simulink model "motion_cue"  (R2015b)
settings: Solver=VariableStepAuto  StartTime=0.0  StopTime=5  FixedStep=.001  MaxStep=.01  RelTol=1e-3
libraries: simulink x1
settings Model: Creator=brownlab  LastModifiedBy=brownlab

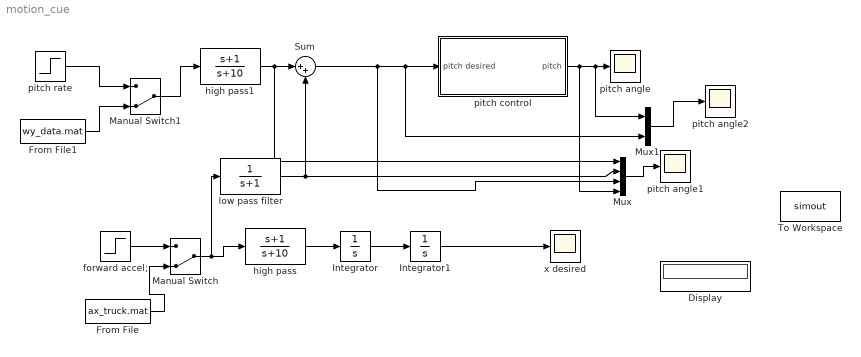
== system motion_cue ==
  Display : Display
  From File : FromFile  FileName=ax_truck.mat  SampleTime=0
  From File1 : FromFile  FileName=wy_data.mat  SampleTime=0
  Integrator : Integrator
  Integrator1 : Integrator
  Manual Switch : ManualSwitch  CurrentSetting=0
  Manual Switch1 : ManualSwitch  CurrentSetting=0
  Mux : Mux
  Mux1 : Mux  Inputs=2
  Sum : Sum  Inputs=|++
  To Workspace : ToWorkspace  VariableName=simout  SaveFormat=Timeseries  SampleTime=-1
  forward accel; : Step  SampleTime=0
  high pass : TransferFcn  Numerator=[1 1]  Denominator=[1 10]
  high pass1 : TransferFcn  Numerator=[1 1]  Denominator=[1 10]
  low pass filter : TransferFcn  Denominator=[1 1]
  pitch angle : Scope
  pitch angle1 : Scope
  pitch angle2 : Scope
  pitch control : Subsystem
  pitch rate : Step  SampleTime=0
  x desired : Scope
  wires:
  pitch control/1(pitch) -> Mux/4, Mux1/1, pitch angle/1
  high pass/1 -> Integrator/1
  Integrator/1 -> Integrator1/1
  Integrator1/1 -> x desired/1
  low pass filter/1 -> Mux/2, Sum/2
  high pass1/1 -> Mux/1, Sum/1
  Sum/1 -> Mux/3, Mux1/2, pitch control/1("pitch desired ")
  Mux/1 -> pitch angle1/1
  forward accel;/1 -> Manual Switch/1
  From File/1 -> Manual Switch/2
  Manual Switch/1 -> low pass filter/1, high pass/1
  pitch rate/1 -> Manual Switch1/1
  From File1/1 -> Manual Switch1/2
  Manual Switch1/1 -> high pass1/1
  Mux1/1 -> pitch angle2/1

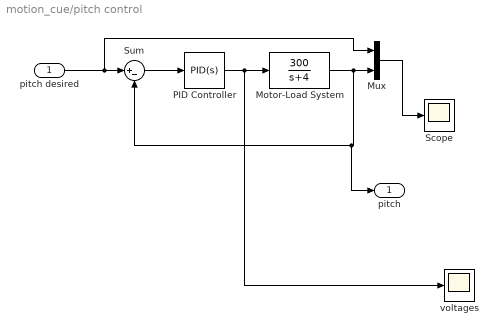
== system motion_cue/pitch control ==
  "pitch desired " : Inport
  Motor-Load System : TransferFcn  Numerator=[300]  Denominator=[1 4]
  Mux : Mux  Inputs=2
  PID Controller : simulink/Continuous/PID Controller  Controller=PID  TimeDomain=Continuous-time  SampleTime=-1  IntegratorMethod=Forward Euler  FilterMethod=Forward Euler  Form=Parallel  UseFilter=on  ControllerParametersSource=internal  P=.1  I=0  D=0  N=100  InitialConditionSource=internal  InitialConditionForIntegrator=0  InitialConditionForFilter=0  ExternalReset=none  LimitOutput=off  UpperSaturationLimit=inf  LowerSaturationLimit=-inf  LinearizeAsGain=on  AntiWindupMode=none  Kb=1  TrackingMode=off  Kt=1  PParamMin=[]  PParamMax=[]  IParamMin=[]  IParamMax=[]  DParamMin=[]  DParamMax=[]  NParamMin=[]  NParamMax=[]  KbParamMin=[]  KbParamMax=[]  KtParamMin=[]  KtParamMax=[]  POutMin=[]  POutMax=[]  IOutMin=[]  IOutMax=[]  DOutMin=[]  DOutMax=[]  NOutMin=[]  NOutMax=[]  KbOutMin=[]  KbOutMax=[]  KtOutMin=[]  KtOutMax=[]  IntegratorOutMin=[]  IntegratorOutMax=[]  FilterOutMin=[]  FilterOutMax=[]  SumOutMin=[]  SumOutMax=[]  SumI1OutMin=[]  SumI1OutMax=[]  SumI2OutMin=[]  SumI2OutMax=[]  SumI3OutMin=[]  SumI3OutMax=[]  SumDOutMin=[]  SumDOutMax=[]  SaturationOutMin=[]  SaturationOutMax=[]  IntegratorContinuousStateAttributes=''  IntegratorStateMustResolveToSignalObject=off  IntegratorRTWStateStorageClass=Auto  FilterContinuousStateAttributes=''  FilterStateMustResolveToSignalObject=off  FilterRTWStateStorageClass=Auto  DifferentiatorICPrevScaledInput=0  DifferentiatorOutMin=[]  DifferentiatorOutMax=[]
  Scope : Scope
  Sum : Sum  Inputs=|+-
  voltages : Scope
  pitch : Outport
  wires:
  PID Controller/1 -> voltages/1, Motor-Load System/1
  "pitch desired "/1 -> Mux/1, Sum/1
  Sum/1 -> PID Controller/1
  Motor-Load System/1 -> pitch/1, Sum/2, Mux/2
  Mux/1 -> Scope/1
